simulink model "Part7"  (R2017b)
settings: Solver=VariableStepAuto  StartTime=0.0  StopTime=100  RelTol=1e-3
settings Model: Creator=Yazdanpanah  LastModifiedBy=admin
settings DataIOCC: ReturnWorkspaceOutputs=on
settings SFSimCC: SimUseLocalCustomCode=on
settings RTWCC: RTWUseLocalCustomCode=on
settings CodeAppCC: StateflowObjectComments=on

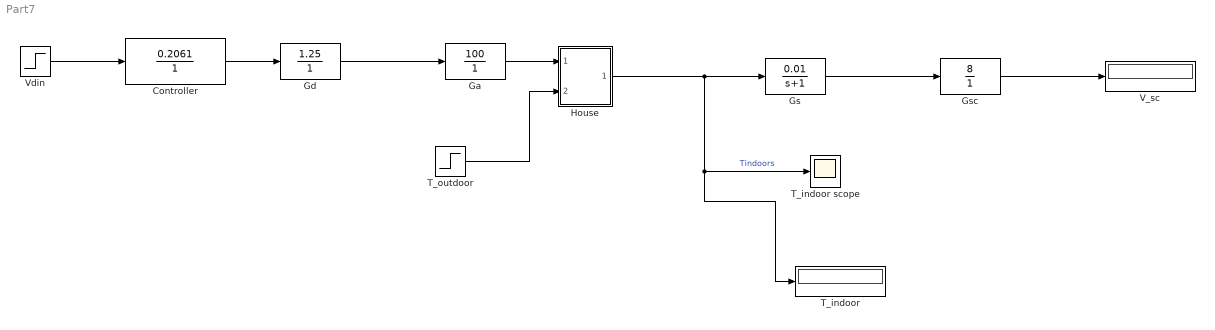
== system Part7 ==
  "Controller " : TransferFcn  Numerator=[0.2061]  Denominator=[1 ]
  Ga : TransferFcn  Numerator=[100]  Denominator=[1 ]
  "Gd " : TransferFcn  Numerator=[1.25]  Denominator=[1 ]
  "Gs " : TransferFcn  Numerator=[0.01]  Denominator=[1 1]
  Gsc : TransferFcn  Numerator=[8]  Denominator=[1 ]
  House : Subsystem
      mask Display: image(fullfile(matlabroot,'toolbox','simulink','simdemos','simgeneral','images','HouseHeatHousePix.svg'))
  "T_indoor " : Display
  "T_indoor scope " : Scope
  T_outdoor : Step  Time=0  After=5  SampleTime=0
  "V_sc " : Display
  "Vdin " : Step  Time=0  After=10  SampleTime=0
  wires:
  "Gd "/1 -> Ga/1
  T_outdoor/1 -> House/2(Outdoor Temp Tout)
  House/1(Room Temp Troom) -> "T_indoor scope "/1, "T_indoor "/1, "Gs "/1  "Tindoors"
  "Gs "/1 -> Gsc/1
  Gsc/1 -> "V_sc "/1
  Ga/1 -> House/1(Heater QDot In)
  "Controller "/1 -> "Gd "/1
  "Vdin "/1 -> "Controller "/1

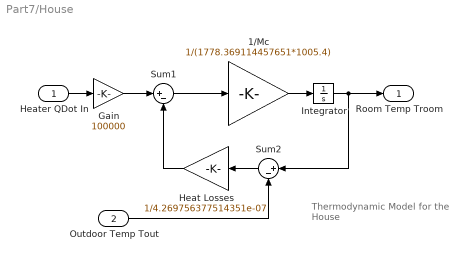
== system Part7/House ==
  note: Thermodynamic Model
      | for the House
  Heater QDot In : Inport
  Outdoor Temp Tout : Inport  Port=2
  1/Mc : Gain  Gain=1/(1778.369114457651*1005.4)  SaturateOnIntegerOverflow=on  OutDataTypeStr=Inherit: Same as input  ParamDataTypeStr=Inherit: Same as input
  Gain : Gain  Gain=100000
  Heat Losses : Gain  Gain=1/4.269756377514351e-07  SaturateOnIntegerOverflow=on  OutDataTypeStr=Inherit: Same as input  ParamDataTypeStr=Inherit: Same as input
  Integrator : Integrator  InitialCondition=20
  Sum1 : Sum  Inputs=|+-  SaturateOnIntegerOverflow=on  InputSameDT=on  OutDataTypeStr=Inherit: Same as first input
  Sum2 : Sum  Inputs=|+-  SaturateOnIntegerOverflow=on  InputSameDT=on  OutDataTypeStr=Inherit: Same as first input
  Room Temp Troom : Outport  InitialOutput=0
  wires:
  Outdoor Temp Tout/1 -> Sum2/2
  Heater QDot In/1 -> Gain/1
  Sum1/1 -> 1/Mc/1
  Sum2/1 -> Heat Losses/1
  Heat Losses/1 -> Sum1/2
  1/Mc/1 -> Integrator/1
  Integrator/1 -> Sum2/1, Room Temp Troom/1
  Gain/1 -> Sum1/1
